simulink model "SIMULINK_SimulationInvertedPendulum"  (R2020a)
settings: Solver=FixedStepAuto  StartTime=0.0  StopTime=30  FixedStep=0.001  RelTol=1e-3
settings Model: Creator=CepaTech  LastModifiedBy=CepaTech

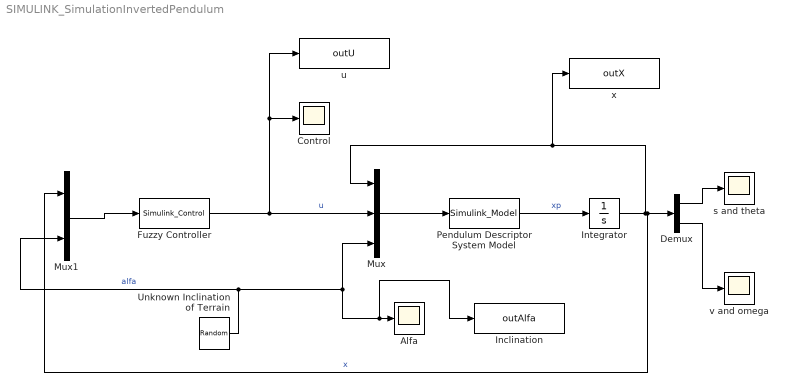
== system SIMULINK_SimulationInvertedPendulum ==
  Alfa : Scope
  Control : Scope
  Demux : Demux  Outputs=2
  Fuzzy Controller : MATLABFcn  MATLABFcn=Simulink_Control
  Inclination : ToWorkspace  VariableName=outAlfa  SampleTime=-1
  Integrator : Integrator  InitialCondition=[0 pi/4 0 0]
  Mux : Mux  Inputs=3
  Mux1 : Mux  Inputs=2
  Pendulum Descriptor System Model : MATLABFcn  MATLABFcn=Simulink_Model
  Unknown Inclination of Terrain : UniformRandomNumber  Minimum=-deg2rad(10)  Maximum=deg2rad(10)  SampleTime=0.5
  s and theta : Scope
  u : ToWorkspace  VariableName=outU  SampleTime=-1
  v and omega : Scope
  x : ToWorkspace  VariableName=outX  SampleTime=-1
  wires:
  Pendulum Descriptor System Model/1 -> Integrator/1  "xp"
  Integrator/1 -> x/1, Mux/1, Demux/1, Mux1/1  "x"
  Demux/1 -> s and theta/1
  Demux/2 -> v and omega/1
  Mux/1 -> Pendulum Descriptor System Model/1
  Fuzzy Controller/1 -> u/1, Control/1, Mux/2  "u"
  Mux1/1 -> Fuzzy Controller/1
  Unknown Inclination of Terrain/1 -> Mux1/2, Mux/3, Inclination/1, Alfa/1  "alfa"
